simulink model "PrinciplePlant"  (R2019b)
settings: Solver=VariableStepAuto  StartTime=0.0  StopTime=10.0  RelTol=1e-3
settings Model: Creator=Lightning  LastModifiedBy=Lightning

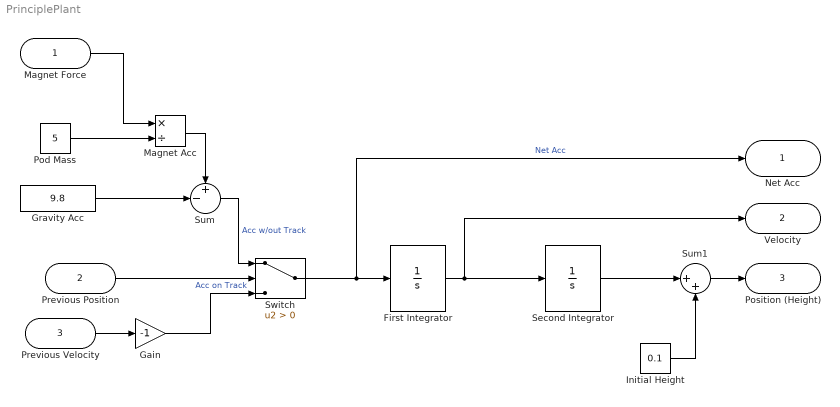
== system PrinciplePlant ==
  Magnet Force : Inport
  Previous Position : Inport  Port=2
  Previous Velocity : Inport  Port=3
  First Integrator : Integrator
  Gain : Gain  Gain=-1
  Gravity Acc : Constant  Value=9.8
  Initial Height : Constant  Value=0.1
  Magnet Acc : Product  Inputs=*/
  Pod Mass : Constant  Value=5
  Second Integrator : Integrator
  Sum : Sum  Inputs=+-|
  Sum1 : Sum  Inputs=|++
  Switch : Switch  Criteria=u2 > Threshold
  Net Acc : Outport
  "Velocity " : Outport  Port=2
  Position (Height) : Outport  Port=3
  wires:
  First Integrator/1 -> Second Integrator/1, "Velocity "/1
  Second Integrator/1 -> Sum1/1
  Magnet Force/1 -> Magnet Acc/1
  Pod Mass/1 -> Magnet Acc/2
  Gravity Acc/1 -> Sum/2
  Magnet Acc/1 -> Sum/1
  Sum/1 -> Switch/1  "Acc w/out Track"
  Gain/1 -> Switch/3  "Acc on Track"
  Switch/1 -> Net Acc/1, First Integrator/1  "Net Acc"
  Previous Velocity/1 -> Gain/1
  Previous Position/1 -> Switch/2
  Sum1/1 -> Position (Height)/1
  Initial Height/1 -> Sum1/2
